simulink model "BrakePedalPressed_plausibility"  (R2024b)
settings: Solver=FixedStepAuto  StartTime=0.0  StopTime=20  RelTol=1e-3
settings Model: Creator=aayan  LastModifiedBy=aayan
settings ConfigComp: CovEnable=on  RecordCoverage=on  CovMetricSettings=dcmwe  CovModelRefEnable=on

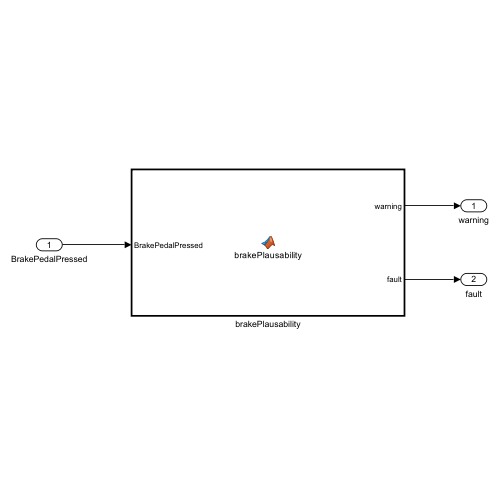
[thumbnail: Simulink's stored preview of the top-level diagram]
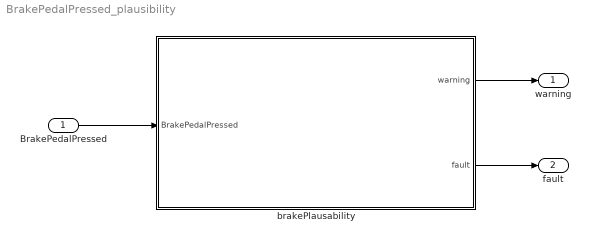
== system BrakePedalPressed_plausibility ==
  BrakePedalPressed : Inport  OutDataTypeStr=boolean
  brakePlausability : MATLAB Function  TreatAsAtomicUnit=on
  warning : Outport
  fault : Outport  Port=2
  wires:
  brakePlausability/1(warning) -> warning/1
  brakePlausability/2(fault) -> fault/1
  BrakePedalPressed/1 -> brakePlausability/1(BrakePedalPressed)

== matlab function BrakePedalPressed_plausibility/brakePlausability ==
  data: BrakePedalPressed input; warning output; fault output
function [warning, fault] = brakePlausability(BrakePedalPressed)

% initialization
warning = boolean(0);
fault =  boolean(0);


if ~islogical(BrakePedalPressed)
    fault = boolean(1);
    warning = boolean(1);
end
